simulink model "moteur_PID_ordre1"  (R2025a)
settings: Solver=VariableStepAuto  StartTime=0.0  StopTime=2  RelTol=1e-3
values from neighbouring files (symbols this model uses):
  K = dcgain(modele)    [Exp.m]
  Ki = omega_n^2/K    [Exp.m]
  Kp = (2*tau/tau_des - 1)/K    [Exp.m]
  tau = -1/p    [Exp.m]
  v_ref = 600    [Exp.m]
settings Model: Creator=vikfo  LastModifiedBy=vikfo

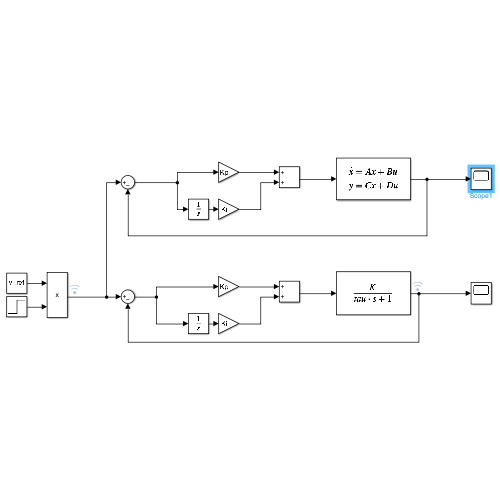
[thumbnail: Simulink's stored preview of the top-level diagram]
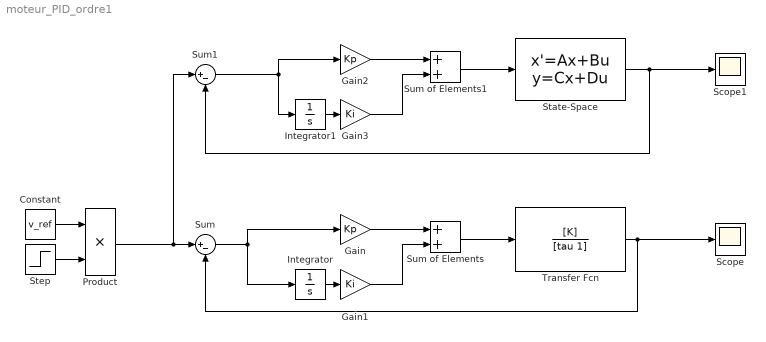
== system moteur_PID_ordre1 ==
  Constant : Constant  Value=v_ref
  Gain : Gain  Gain=Kp
  Gain1 : Gain  Gain=Ki
  Gain2 : Gain  Gain=Kp
  Gain3 : Gain  Gain=Ki
  Integrator : Integrator
  Integrator1 : Integrator
  Product : Product
  Scope : Scope
      settings: ActiveDisplayYMinimum=-1482.8201061777609  ActiveDisplayYMaximum=4014.9462502557749
  Scope1 : Scope
      settings: ActiveDisplayYMinimum=144.84841564320209  ActiveDisplayYMaximum=694.65780540710909
  State-Space : StateSpace  A=[0 1; 0 -1/tau]  B=[0; K/tau]  C=[0 1]  D=0  InitialCondition=0
  Step : Step  Time=0  SampleTime=0
  Sum : Sum  Inputs=|+-
  Sum of Elements : Sum
  Sum of Elements1 : Sum
  Sum1 : Sum  Inputs=|+-
  Transfer Fcn : TransferFcn  Numerator=[K]  Denominator=[tau 1]
  wires:
  Product/1 -> Sum1/1, Sum/1
  Integrator/1 -> Gain1/1
  Sum/1 -> Integrator/1, Gain/1
  Sum of Elements/1 -> Transfer Fcn/1
  Gain/1 -> Sum of Elements/1
  Gain1/1 -> Sum of Elements/2
  Transfer Fcn/1 -> Sum/2, Scope/1
  Constant/1 -> Product/1
  Step/1 -> Product/2
  Gain2/1 -> Sum of Elements1/1
  State-Space/1 -> Sum1/2, Scope1/1
  Sum of Elements1/1 -> State-Space/1
  Sum1/1 -> Integrator1/1, Gain2/1
  Gain3/1 -> Sum of Elements1/2
  Integrator1/1 -> Gain3/1
